simulink model "PVTOL_SMC_Chattering_20204b"  (R2024b)
settings: Solver=ode4  StartTime=0.0  StopTime=50  FixedStep=0.0001  RelTol=1e-3
settings Model: Creator=nestorhernandezcastellanos  LastModifiedBy=nestorhernandezcastellanos
settings ModelReferenceCC: UpdateModelReferenceTargets=IfOutOfDate
settings SFSimCC: SimGPUStackLimitPerThread=51200
settings RTWCC: GPUStackLimitPerThread=51200  GPUComputeCapability=7.5
settings ConfigComp: CovMetricSettings=de  CovBoundaryAbsTol=1.0e-5

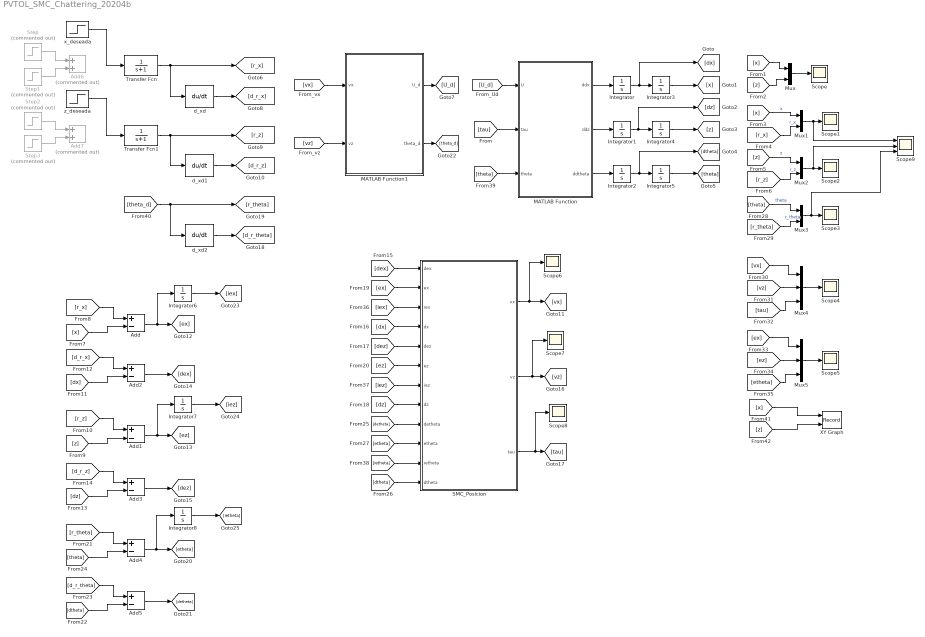
== system PVTOL_SMC_Chattering_20204b ==
  Add{,1..5} (6 alike) : Sum  Inputs=+-
  Add6 : Sum  Commented=on
  Add7 : Sum  Commented=on
  Integrator{,1..8} (9 alike) : Integrator
  MATLAB Function : MATLAB Function  TreatAsAtomicUnit=on
  MATLAB Function1 : MATLAB Function  TreatAsAtomicUnit=on
  Mux{,1..3} (4 alike) : Mux  Inputs=2
  Mux4 : Mux  Inputs=3
  Mux5 : Mux  Inputs=3
  SMC_Posicion : MATLAB Function  TreatAsAtomicUnit=on
  Scope{,1..8} (9 alike) : Scope
  Scope9 : Scope  NumInputPorts=3
  Step : Step  Commented=on  After=3  SampleTime=0
  Step1 : Step  Commented=on  Time=15  After=7  SampleTime=0
  Step2 : Step  Commented=on  After=3  SampleTime=0
  Step3 : Step  Commented=on  Time=15  After=7  SampleTime=0
  Transfer Fcn : TransferFcn  Denominator=[1 1]
  Transfer Fcn1 : TransferFcn  Denominator=[1 1]
  XY Graph : Record  FileSettingsInternal="{\"entries\":[{\"content\":{\"excelSettings\":{\"content\":{},\"type\":\"Streamout.ExcelSettings\"},\"parquetSettings\":{\"content\":{},\"type\":\"Streamout.ParquetSettings\"}},\"type\":\"Streamout.FileSettingStorage\",\"uuid\":\"\"}],\"packageUris\":[\"http:\\/\\/schema.mathworks.com\\/mf0\\/streamout_blocks\\/R2020a\"],\"version\":\"1.0\"}"  Layout=[1 1]  SignalsInternal="{\"entries\":[{\"content\":{\"signals\":[{\"content\":{\"blockPath\":[],\"dimensions\":[1],\"domain\":\"\",\"lineColor\":\"#a2142f\",\"plots\":[ 1 ],\"port\":1,\"signalID\":1,\"signalName\":\"From41\"},\"type\":\"RecordBlkView.Signal\",\"uuid\":\"\"},{\"content\":{\"blockPath\":[],\"dimensions\":[1],\"domain\":\"\",\"lineColor\":\"#139fff\",\"plots\":[ 1 ],\"port\":2,\"signalID\":2,\"signalName\":\"From42\"},\"type\":\"RecordBlkView.Signal\",\"uuid\":\"\"}]},\"type\":\"RecordBlkView.InputSignals\",\"uuid\":\"\"}],\"packageUris\":[\"http:\\/\\/schema.mathworks.com\\/mf0\\/streamout_blocks\\/R2020a\"],\"version\":\"1.0\"}"  VisualizationBindings="{\"xyplotplugin\":{\"info\":[{\"series\":[{\"bindingParametersList\":[{\"parameter\":\"X-Axis\",\"signalID\":1,\"signalName\":\"From41\"},{\"parameter\":\"Y-Axis\",\"signalID\":2,\"signalName\":\"From42\"}],\"seriesID\":0}],\"subplotID\":1}]}}"  CompatibilityTag=XY
  d_xd : Derivative
  d_xd1 : Derivative
  d_xd2 : Derivative
  x_deseada : Step  After=5  SampleTime=0
  z_deseada : Step  After=5  SampleTime=0
  wires:
  Mux/1 -> Scope/1
  [z] -> Mux/2
  [x] -> Mux/1
  [x] -> Mux1/1  "x"
  [r_x] -> Mux1/2  "r_x"
  [r_z] -> Mux2/2  "r_z"
  [z] -> Mux2/1  "z"
  [r_x] -> Add/1
  [x] -> Add/2
  Add/1 -> Integrator6/1, [ex]
  [z] -> Add1/2
  [r_z] -> Add1/1
  Add2/1 -> [dex]
  [dx] -> Add2/2
  [d_r_x] -> Add2/1
  [d_r_z] -> Add3/1
  [dz] -> Add3/2
  Add3/1 -> [dez]
  SMC_Posicion/1(vx) -> Scope6/1, [vx]
  SMC_Posicion/2(vz) -> Scope7/1, [vz]
  SMC_Posicion/3(tau) -> Scope8/1, [tau]
  [dex] -> SMC_Posicion/1(dex)
  [dx] -> SMC_Posicion/4(dx)
  [dez] -> SMC_Posicion/5(dez)
  [dz] -> SMC_Posicion/8(dz)
  [ex] -> SMC_Posicion/2(ex)
  [ez] -> SMC_Posicion/6(ez)
  Add5/1 -> [detheta]
  [dtheta] -> Add5/2
  [d_r_theta] -> Add5/1
  [r_theta] -> Add4/1
  [theta] -> Add4/2
  [detheta] -> SMC_Posicion/9(detheta)
  [etheta] -> SMC_Posicion/10(etheta)
  [dtheta] -> SMC_Posicion/12(dtheta)
  [theta] -> Mux3/1  "theta"
  [r_theta] -> Mux3/2  "r_theta"
  Mux4/1 -> Scope4/1
  [vz] -> Mux4/2
  [vx] -> Mux4/1
  [tau] -> Mux4/3
  [etheta] -> Mux5/3
  [ex] -> Mux5/1
  [ez] -> Mux5/2
  Mux5/1 -> Scope5/1
  [iex] -> SMC_Posicion/3(iex)
  [iez] -> SMC_Posicion/7(iez)
  [ietheta] -> SMC_Posicion/11(ietheta)
  Integrator6/1 -> [iex]
  Integrator7/1 -> [iez]
  Add1/1 -> Integrator7/1, [ez]
  Add4/1 -> Integrator8/1, [etheta]
  Integrator8/1 -> [ietheta]
  x_deseada/1 -> Transfer Fcn/1
  Integrator3/1 -> [x]
  z_deseada/1 -> Transfer Fcn1/1
  [tau] -> MATLAB Function/2(tau)
  Step1/1 -> Add6/2
  MATLAB Function1/1(U_d) -> [U_d]
  Step/1 -> Add6/1
  Step2/1 -> Add7/1
  Integrator5/1 -> [theta]
  Transfer Fcn1/1 -> d_xd1/1, [r_z]
  [theta_d] -> [r_theta], d_xd2/1
  Step3/1 -> Add7/2
  MATLAB Function/2(ddz) -> Integrator1/1
  Integrator1/1 -> [dz], Integrator4/1
  d_xd/1 -> [d_r_x]
  MATLAB Function/3(ddtheta) -> Integrator2/1
  [U_d] -> MATLAB Function/1(U)
  [vz] -> MATLAB Function1/2(vz)
  [vx] -> MATLAB Function1/1(vx)
  MATLAB Function1/2(theta_d) -> [theta_d]
  Transfer Fcn/1 -> [r_x], d_xd/1
  d_xd2/1 -> [d_r_theta]
  Integrator2/1 -> [dtheta], Integrator5/1
  [theta] -> MATLAB Function/3(theta)
  MATLAB Function/1(ddx) -> Integrator/1
  Integrator4/1 -> [z]
  d_xd1/1 -> [d_r_z]
  Integrator/1 -> [dx], Integrator3/1
  Mux1/1 -> Scope9/1, Scope1/1
  Mux3/1 -> Scope9/3, Scope3/1
  Mux2/1 -> Scope9/2, Scope2/1
  [z] -> XY Graph/2
  [x] -> XY Graph/1

== matlab function PVTOL_SMC_Chattering_20204b/MATLAB Function1 ==
  data: vx input; U_d output; vz input; theta_d output
function [U_d,theta_d] = linealizacion(vx,vz)

g = 9.81;                                  
U_d = sqrt(vx^2 + (vz+g)^2);                 
theta_d = atan2(-vx,vz+g);

== matlab function PVTOL_SMC_Chattering_20204b/MATLAB Function ==
  data: U input; ddx output; tau input; theta input; ddz output; ddtheta output
function [ddx,ddz,ddtheta] = planta(U,tau,theta)

g = 9.81;                                       

ddx = -U*sin(theta);                            
ddz = U*cos(theta)-g;                           
ddtheta = tau;

== matlab function PVTOL_SMC_Chattering_20204b/SMC_Posicion ==
  data: dex input; ex input; iex input; dx input; vx output; dez input; ez input; iez input; dz input; vz output; tau output; detheta input; etheta input; ietheta input; dtheta input
function [vx, vz, tau] = controlador(dex, ex, iex, dx, dez, ez, iez, dz, detheta, etheta, ietheta, dtheta)

% Ganancias del controlador
Kx = 1.65;
Kz = 1.75;
Ktheta = 1.35;

% Superficies integrales
mx1 = 0.215;
mx2 = 0.0295;

mz1 = 0.55;
mz2 = 0.90;

mtheta1 = 1.10;
mtheta2 = 0.15;

% Cotas
Lx = 0.225;
Lz = 0.75;
Ltheta = 0.75;

% Superficies de deslizamiento integrales
sigma_x = dex + mx1*ex + mx2*iex;
sigma_z = dez + mz1*ez + mz2*iez;
sigma_theta = detheta + mtheta1*etheta + mtheta2*ietheta;

% Valores equivalentes
Veq_x = Lx + mx1*abs(dx) + mx2*abs(ex);
Veq_z = Lz + mz1*abs(dz) + mz2*abs(ez);
Veq_theta = Ltheta + mtheta1*abs(dtheta) + mtheta2*abs(etheta);

% Leyes de control
vx = Kx*Veq_x*sign(sigma_x);
vz = Kz*Veq_z*sign(sigma_z);
tau = Ktheta*Veq_theta*sign(sigma_theta);
